simulink model "wireless"  (Simulink 4.00)
settings: Solver=ode45  StartTime=0.0  StopTime=10  RelTol=1e-3
InitFcn:
  | clear functions
undefined symbols (not defined in the file or in its folder): WLAN
libraries: truetime x3
settings Model: Creator=anton  LastModifiedBy=anton  SaveTime=off  SaveOutput=off  RTWOptions="-aEnforceIntegerDowncast=1 -aFoldNonRolledExpr=1 -aInlineInvariantSignals=0 -aInlineParameters=0 -aLocalBlockOutputs=1 -aRollThreshold=5 -aGenerateReport=0 -aGenCodeOnly=0 -aRTWVerbose=1 -aIncludeHyperlinkInReport=0 -aLaunchReport=0 -aForceParamTrailComments=0 -aGenerateComments=1 -aIgnoreCustomStorageClasses=1 -aIncHierarchyInIds=0 -aMaxRTWIdLen=31 -aShowEliminatedStatements=0 -aPrefixModelToSubsysFcnNames=1 -aIncDataTypeInIds=0 -aInsertBlockDesc=0 -aSimulinkBlockComments=1 -aInlinedPrmAccess=\"Literals\"  -aSuppressErrorStatus=0 -aModelReferenceCompliant=1 -aSupportNonInlinedSFcns=1 -aSupportContinuousTime=1 -aSupportComplex=1 -aSupportNonFinite=1 -aSupportAbsoluteTime=1 -aTargetPreCompLibLocation=\"\" -aTargetLibSuffix=\"\" -aTargetFcnLib=\"ansi_tfl_tmw.mat\" -aMultiInstanceERTCode=0 -aLogVarNameModifier=\"rt_\" -aIsPILTarget=0 -aCombineOutputUpdateFcns=0 -aGenerateASAP2=0 -aGenerateSampleERTMain=0 -aGenerateFullHeader=1 -aUtilityFuncGeneration=\"Auto\" -aIncludeFileDelimiter=\"Auto\" -aIncludeMdlTerminateFcn=1 -aPurelyIntegerCode=0 -aERTCustomFileBanners=0 -aRTWCAPIStates=0 -aRTWCAPIParams=0 -aRTWCAPISignals=0 -aMatFileLogging=1 -aGenFloatMathFcnCalls=\"ANSI_C\" -aExtModeMexFile=\"ext_comm\" -aExtModeTransport=0 -aExtModeStaticAllocSize=1000000 -aExtModeTesting=0 -aExtModeStaticAlloc=0 -aExtMode=0"  ExtModeAutoUpdateStatusClock=off  BlockReductionOpt=off

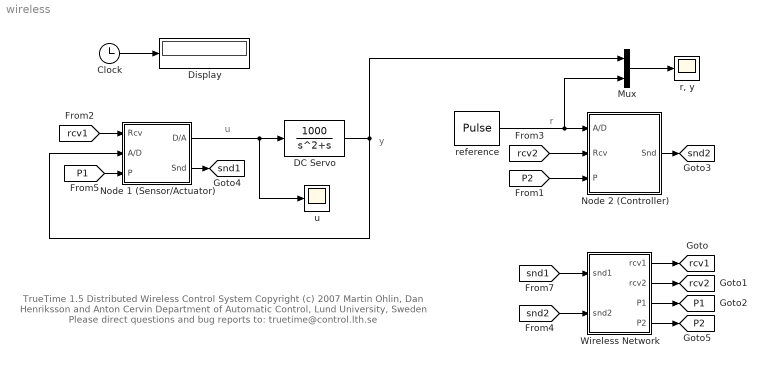
== system wireless ==
  note: u
  note: y
  note: r
  note: TrueTime 1.5  Distributed Wireless Control System
      | Copyright (c) 2007
      | Martin Ohlin, Dan Henriksson and Anton Cervin
      | Department of Automatic Control, Lund University, Sweden
      | Please direct questions and bug reports to:  truetime@control.lth.se
  Clock : Clock
      settings: DisplayTime=off  Decimation=10
  DC Servo : TransferFcn  Numerator=[1000]  Denominator=[1 1 0]  AbsoluteTolerance=auto  Realization=auto
  Display : Display
      settings: Format=short
  Mux : Mux  Inputs=2
  Node 1 (Sensor/Actuator) : Subsystem
      settings: RTWFcnNameOpts=Auto  RTWFileNameOpts=Auto
  Node 2 (Controller) : Subsystem
      settings: RTWFcnNameOpts=Auto  RTWFileNameOpts=Auto
  Wireless Network : Subsystem
      settings: RTWFcnNameOpts=Auto  RTWFileNameOpts=Auto
  "r, y" : Scope
      settings: TimeRange=10  YMin=-0.717285  YMax=1.85596  SaveToWorkspace=off  SaveName=y  MaxDataPoints=5000
  reference : DiscretePulseGenerator  PulseType=Time-based  Amplitude=1  Period=1.2  PulseWidth=50  PhaseDelay=0  SampleTime=1
  u : Scope
      settings: TimeRange=10  YMin=-2  YMax=6  SaveToWorkspace=off  SaveName=u  MaxDataPoints=5000
  tag scope: P1=global, P2=global, rcv1=global, rcv2=global, snd1=global, snd2=global
  wires:
  [snd1] -> Wireless Network/1(snd1)
  Wireless Network/1(rcv1) -> [rcv1]
  Node 1 (Sensor/Actuator)/1(D/A) -> DC Servo/1, u/1
  Node 2 (Controller)/1(Snd) -> [snd2]
  [rcv1] -> Node 1 (Sensor/Actuator)/1(Rcv)
  Clock/1 -> Display/1
  reference/1 -> Node 2 (Controller)/1(A/D), Mux/2
  Wireless Network/2(rcv2) -> [rcv2]
  [rcv2] -> Node 2 (Controller)/2(Rcv)
  Mux/1 -> "r, y"/1
  DC Servo/1 -> Mux/1, Node 1 (Sensor/Actuator)/2(A/D)
  Node 1 (Sensor/Actuator)/2(Snd) -> [snd1]
  [snd2] -> Wireless Network/2(snd2)
  Wireless Network/4(P2) -> [P2]
  Wireless Network/3(P1) -> [P1]
  [P2] -> Node 2 (Controller)/3(P)
  [P1] -> Node 1 (Sensor/Actuator)/3(P)

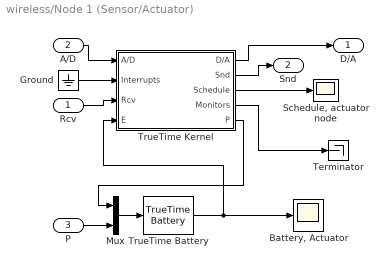
== system wireless/Node 1 (Sensor/Actuator) ==
  Rcv : Inport  Port=1  LatchInput=off
  A/D : Inport  Port=2  LatchInput=off
  P : Inport  Port=3  LatchInput=off
  "Battery, Actuator" : Scope
      settings: TimeRange=10  YMin=0  YMax=0.3  SaveToWorkspace=off  MaxDataPoints=5000
  Ground : Ground
  Mux : Mux  Inputs=2
  "Schedule, actuator node" : Scope
      settings: TickLabels=on  TimeRange=10  YMin=1  YMax=6  SaveToWorkspace=off  SaveName=ScopeData  DataFormat=Array  MaxDataPoints=5000
  Terminator : Terminator
  TrueTime Battery : truetime/TrueTime Battery  energy=0.3
  TrueTime Kernel : Subsystem  AncestorBlock=truetime/TrueTime Kernel  mask{sfun=actuator_init, args=0, battery=on, clockdrift=0, clockoffset=0}
      mask prompts: sfun "Name of init function (MEX or MATLAB)"; args "Init function argument"; clockdrift "Clock drift"; clockoffset "Clock offset"
      settings: RTWFcnNameOpts=Auto  RTWFileNameOpts=Auto
      mask CallbackString: ||batterychange||
  D/A : Outport  Port=1
  Snd : Outport  Port=2
  wires:
  A/D/1 -> TrueTime Kernel/1(A/D)
  Rcv/1 -> TrueTime Kernel/3(Rcv)
  Ground/1 -> TrueTime Kernel/2(Interrupts)
  TrueTime Kernel/1(D/A) -> D/A/1
  TrueTime Kernel/2(Snd) -> Snd/1
  TrueTime Kernel/3(Schedule) -> "Schedule, actuator node"/1
  TrueTime Kernel/4(Monitors) -> Terminator/1
  Mux/1 -> TrueTime Battery/1
  P/1 -> Mux/2
  TrueTime Kernel/5(P) -> Mux/1
  TrueTime Battery/1 -> "Battery, Actuator"/1, TrueTime Kernel/4(E)

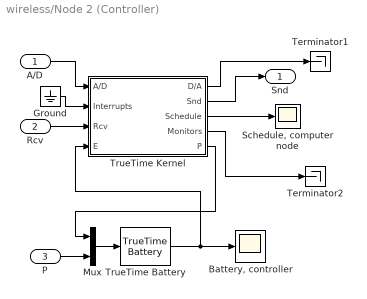
== system wireless/Node 2 (Controller) ==
  A/D : Inport  Port=1  LatchInput=off
  Rcv : Inport  Port=2  LatchInput=off
  P : Inport  Port=3  LatchInput=off
  "Battery, controller" : Scope
      settings: TimeRange=10  YMin=0  YMax=0.3  SaveToWorkspace=off  SaveName=ScopeData2  MaxDataPoints=5000
  Ground : Ground
  Mux : Mux  Inputs=2
  "Schedule, computer node" : Scope
      settings: TimeRange=10  YMin=1  YMax=5  SaveName=schedule  MaxDataPoints=5000
  Terminator1 : Terminator
  Terminator2 : Terminator
  TrueTime Battery : truetime/TrueTime Battery  energy=0.3
  TrueTime Kernel : Subsystem  AncestorBlock=truetime/TrueTime Kernel  mask{sfun=controller_init, args=0, battery=on, clockdrift=0, clockoffset=0}
      mask prompts: sfun "Name of init function (MEX or MATLAB)"; args "Init function argument"; clockdrift "Clock drift"; clockoffset "Clock offset"
      settings: RTWFcnNameOpts=Auto  RTWFileNameOpts=Auto
      mask CallbackString: ||batterychange||
  Snd : Outport  Port=1
  wires:
  TrueTime Kernel/2(Snd) -> Snd/1
  Ground/1 -> TrueTime Kernel/2(Interrupts)
  A/D/1 -> TrueTime Kernel/1(A/D)
  Rcv/1 -> TrueTime Kernel/3(Rcv)
  TrueTime Kernel/3(Schedule) -> "Schedule, computer node"/1
  TrueTime Kernel/1(D/A) -> Terminator1/1
  Mux/1 -> TrueTime Battery/1
  P/1 -> Mux/2
  TrueTime Kernel/5(P) -> Mux/1
  TrueTime Kernel/4(Monitors) -> Terminator2/1
  TrueTime Battery/1 -> "Battery, controller"/1, TrueTime Kernel/4(E)

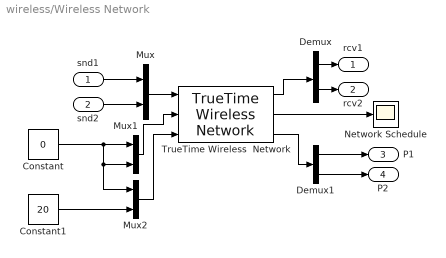
== system wireless/Wireless Network ==
  snd1 : Inport  Port=1  LatchInput=off
  snd2 : Inport  Port=2  LatchInput=off
  Constant : Constant  Value=0
  Constant1 : Constant  Value=20
  Demux : Demux  Outputs=2  BusSelectionMode=off
  Demux1 : Demux  Outputs=2  BusSelectionMode=off
  Mux : Mux  Inputs=2
  Mux1 : Mux  Inputs=2
  Mux2 : Mux  Inputs=2
  Network Schedule : Scope
      settings: TimeRange=10  YMin=1  YMax=2.5  SaveName=nschedule  MaxDataPoints=5000
  TrueTime Wireless  Network : truetime/TrueTime Wireless  Network  nwtype=802.11b (WLAN)  nwnbr=1  nnodes=2  rate=800000  minsize=272  transpower=20  threshold=-48  pathloss=3.5  use_pathloss_function=off  acktimeout=0.00004  retrylimit=5  error_threshold=0.03
  rcv1 : Outport  Port=1
  rcv2 : Outport  Port=2
  P1 : Outport  Port=3
  P2 : Outport  Port=4
  wires:
  Demux/1 -> rcv1/1
  Demux/2 -> rcv2/1
  snd1/1 -> Mux/1
  snd2/1 -> Mux/2
  TrueTime Wireless  Network/1 -> Demux/1
  TrueTime Wireless  Network/2 -> Network Schedule/1
  Mux/1 -> TrueTime Wireless  Network/1
  TrueTime Wireless  Network/3 -> Demux1/1
  Mux2/1 -> TrueTime Wireless  Network/3
  Mux1/1 -> TrueTime Wireless  Network/2
  Demux1/1 -> P1/1
  Demux1/2 -> P2/1
  Constant/1 -> Mux1/1, Mux1/2, Mux2/1
  Constant1/1 -> Mux2/2

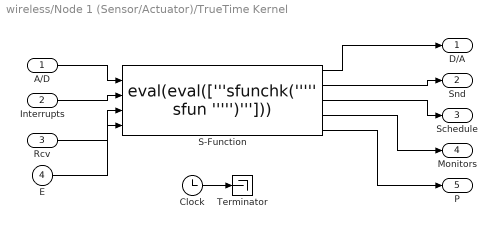
== system wireless/Node 1 (Sensor/Actuator)/TrueTime Kernel ==
  A/D : Inport  Port=1  LatchInput=off
  Interrupts : Inport  Port=2  LatchInput=off
  Rcv : Inport  Port=3  LatchInput=off
  E : Inport  Port=4  LatchInput=off
  Clock : Clock
      settings: DisplayTime=off  Decimation=10
  S-Function : S-Function  FunctionName=eval(eval(['''sfunchk(''''' sfun ''''')''']))  Parameters=sfun, args, clockdrift, clockoffset  PortCounts=[]  SFunctionModules=''
  Terminator : Terminator
  D/A : Outport  Port=1
  Snd : Outport  Port=2
  Schedule : Outport  Port=3
  Monitors : Outport  Port=4
  P : Outport  Port=5
  wires:
  Clock/1 -> Terminator/1
  Rcv/1 -> S-Function/3
  Interrupts/1 -> S-Function/2
  S-Function/4 -> Monitors/1
  S-Function/3 -> Schedule/1
  S-Function/1 -> D/A/1
  S-Function/2 -> Snd/1
  A/D/1 -> S-Function/1
  E/1 -> S-Function/4
  S-Function/5 -> P/1

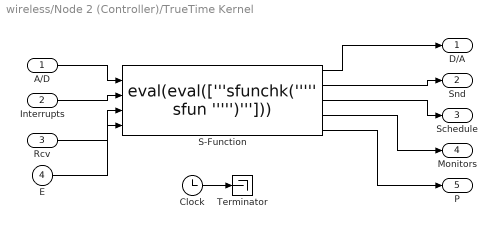
== system wireless/Node 2 (Controller)/TrueTime Kernel ==
  A/D : Inport  Port=1  LatchInput=off
  Interrupts : Inport  Port=2  LatchInput=off
  Rcv : Inport  Port=3  LatchInput=off
  E : Inport  Port=4  LatchInput=off
  Clock : Clock
      settings: DisplayTime=off  Decimation=10
  S-Function : S-Function  FunctionName=eval(eval(['''sfunchk(''''' sfun ''''')''']))  Parameters=sfun, args, clockdrift, clockoffset  PortCounts=[]  SFunctionModules=''
  Terminator : Terminator
  D/A : Outport  Port=1
  Snd : Outport  Port=2
  Schedule : Outport  Port=3
  Monitors : Outport  Port=4
  P : Outport  Port=5
  wires:
  Clock/1 -> Terminator/1
  Rcv/1 -> S-Function/3
  Interrupts/1 -> S-Function/2
  S-Function/4 -> Monitors/1
  S-Function/3 -> Schedule/1
  S-Function/1 -> D/A/1
  S-Function/2 -> Snd/1
  A/D/1 -> S-Function/1
  E/1 -> S-Function/4
  S-Function/5 -> P/1
